simulink model "SimulationLinear"  (Simulink 9.2)
settings: Solver=ode1  StartTime=0.0  StopTime=30  FixedStep=T  RelTol=1e-3  EnableMultiTasking=on
values from neighbouring files (symbols this model uses):
  A = [zeros(2,2),    eye(2,2) ... (first row only)    [StateFeedback_Controller_Observer_Design.m]    (also in equilibriumpositon_2_realsim.mat = [0 0 1.86000056553 -118.859256664 0 0 -4.86792536172 -131.56)
  B = [zeros(2,2) ... (first row only)    [StateFeedback_Controller_Observer_Design.m]    (also in equilibriumpositon_2_realsim.mat = [0 0 0.0946459156765 0.178753935587])
  C = [h*q2dot   h*(q1dot+q2dot) ... (first row only)    [NonLinModel.m]    (also in StateFeedback_Controller_Observer_Design.m = [1 0 0 0; equilibriumpositon_2_realsim.mat = [1  0  0  0; 0  1  0  0])
  K = place(A,B,p)    [StateFeedback_Controller_Observer_Design.m]    (also in equilibriumpositon_2_realsim.mat = [3103.64468197 1789.25362632 433.04949119 3.48374472995])
  L = transpose(place(A', C',po))    [StateFeedback_Controller_Observer_Design.m]    (also in equilibriumpositon_2_realsim.mat = [220.529108681  -24.0242041595; -32.2456951439  226.07999002)
  q1 = x(1)    [NonLinModel.m]    (also in StateFeedback_Controller_Observer_Design.m = 1.57079632679; equilibriumpositon_2_realsim.mat = 1.57079632679)
  q2 = x(2)    [NonLinModel.m]    (also in StateFeedback_Controller_Observer_Design.m = 0; equilibriumpositon_2_realsim.mat = 3.14159265359)
  T = .001    (= 0.001)    [StateFeedback_Controller_Observer_Design.m]    (also in equilibriumpositon_2_realsim.mat)
  X0 = [q1+.1 q2-.2 0 0]    [StateFeedback_Controller_Observer_Design.m]    (also in equilibriumpositon_2_realsim.mat = [1.67079632679 2.94159265359 0 0])
undefined symbols (not defined in the file or in its folder): DiscIntNeverNeededParam
settings Model: Creator=jafarm2  LastModifiedBy=AndyA  ExtModeTrigDuration=5000
settings SolverCC: PositivePriorityOrder=on
settings OptimizationCC: ExpressionDepthLimit=2147483647
settings DebuggingCC: SolverPrmCheckMsg=warning
settings RTWCC: SystemTargetFile=quarc_win64.tlc  TemplateMakefile=quarc_default_tmf  Description=QUARC Win64 Target
settings STFCustomTargetCC: TargetPreCompLibLocation=C:\PROGRA~3\QUARC\lib\2011b\win64\release  GeneratePreprocessorConditionals=Disable all  CPPClassGenCompliant=on  SystemTargetFile=quarc_win64.tlc
settings GRTTargetCC: TargetPreCompLibLocation=C:\PROGRA~3\QUARC\lib\2011b\win64\release  ParMdlRefBuildCompliant=off  CompOptLevelCompliant=off  ConcurrentExecutionCompliant=off  MatFileLogging=off  UseToolchainInfoCompliant=off  ExtMode=on  ExtModeMexFile=quarc_comm

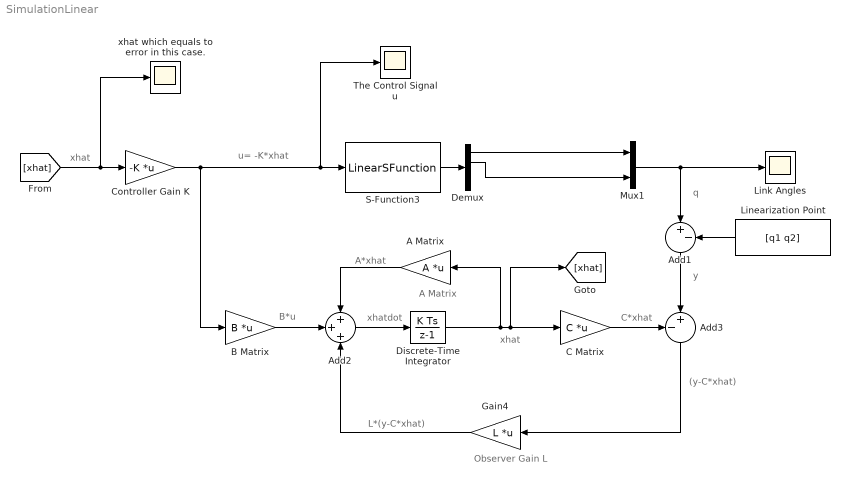
== system SimulationLinear ==
  note: q
  note: y
  note: B*u
  note: A Matrix
  note: A*xhat
  note: xhat
  note: C*xhat
  note: (y-C*xhat)
  note: L*(y-C*xhat)
  note: Observer Gain L
  note: u= -K*xhat
  note: xhat
  note: xhatdot
  A Matrix : Gain  Gain=A  Multiplication=Matrix(K*u)
  Add1 : Sum  Inputs=|+-
  Add2 : Sum  Inputs=+++
  Add3 : Sum  Inputs=-+|
  B Matrix : Gain  Gain=B  Multiplication=Matrix(K*u)
  C Matrix : Gain  Gain=C  Multiplication=Matrix(K*u)
  Controller Gain K : Gain  Gain=-K  Multiplication=Matrix(K*u)
  Demux : Demux
  Discrete-Time Integrator : DiscreteIntegrator  InitialCondition=[0 0 0 0]'  SampleTime=T  ICPrevOutput=DiscIntNeverNeededParam  ICPrevScaledInput=DiscIntNeverNeededParam
  Gain4 : Gain  Gain=L  Multiplication=Matrix(K*u)
  Linearization Point : Constant  Value=[q1 q2]
  Link Angles : Scope
  Mux1 : Mux  Inputs=2
  S-Function3 : S-Function  FunctionName=LinearSFunction  Parameters=X0,A,B,C  SFunctionDeploymentMode=off  EnableBusSupport=off
  The Control Signal u : Scope
  xhat which equals to error in this case. : Scope
  wires:
  Controller Gain K/1 -> B Matrix/1, The Control Signal u/1, S-Function3/1
  Mux1/1 -> Link Angles/1, Add1/1
  Demux/1 -> Mux1/1
  Demux/2 -> Mux1/2
  Add2/1 -> Discrete-Time Integrator/1
  C Matrix/1 -> Add3/1
  Add3/1 -> Gain4/1
  Discrete-Time Integrator/1 -> A Matrix/1, C Matrix/1, [xhat]
  B Matrix/1 -> Add2/2
  A Matrix/1 -> Add2/1
  Add1/1 -> Add3/2
  Linearization Point/1 -> Add1/2
  Gain4/1 -> Add2/3
  [xhat] -> Controller Gain K/1, xhat which equals to error in this case./1
  S-Function3/1 -> Demux/1
